simulink model "Potoo_Dyn_Model_v3px4_Flap_compact"  (R2024b)
settings: Solver=FixedStepAuto  StartTime=0.0  StopTime=120  FixedStep=0.001  MaxStep=0.001  RelTol=1e-3
InitFcn:
  | Tmech = 0.004;
undefined symbols (not defined in the file): Control, custom_ff, DiscIntNeverNeededParam, Earth, F, fractalcoef, Light, MIL, Potoo, Px4_Parms, realflap, tau, theta_max, thetadot_max, WGS84
libraries: cstblocks x10, matrix_library x10, aerolibasang x7, simulink x6, aerolibadyn x3, sharedtransform x2, slctrl_autotuning x1, mspfiltlib x1, mspsensorlib x1, shared6dof x1, aerolibactuator x1, aerolibatmos2 x1
(part 1 of 2)
settings Model: Creator=antho  LastModifiedBy=Nathan
settings SolverCC: AutoInsertRateTranBlk=on

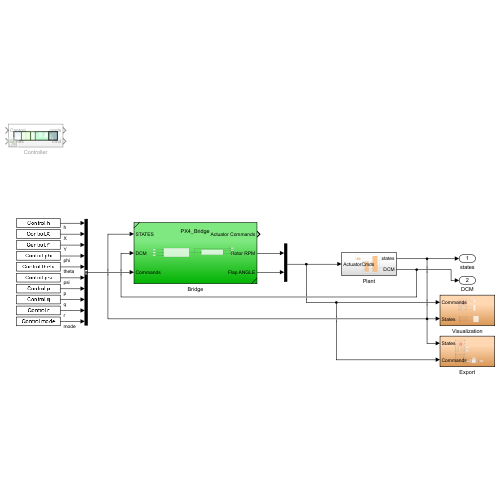
[thumbnail: Simulink's stored preview of the top-level diagram]
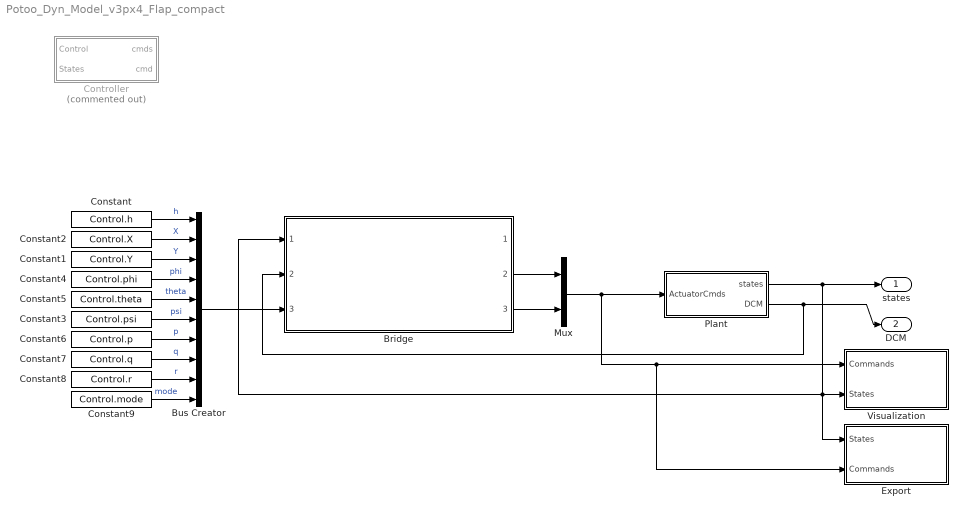
== system Potoo_Dyn_Model_v3px4_Flap_compact ==
  Bridge : Subsystem  ReferencedSubsystem=PX4_Bridge
  Bus Creator : BusCreator  Inputs=10
  Constant : Constant  Value=Control.h
  Constant1 : Constant  Value=Control.Y
  Constant2 : Constant  Value=Control.X
  Constant3 : Constant  Value=Control.psi
  Constant4 : Constant  Value=Control.phi
  Constant5 : Constant  Value=Control.theta
  Constant6 : Constant  Value=Control.p
  Constant7 : Constant  Value=Control.q
  Constant8 : Constant  Value=Control.r
  Constant9 : Constant  Value=Control.mode
  Controller : Subsystem  Commented=on
  Export : Subsystem
  Mux : Mux  Inputs=2
  Plant : Subsystem
  Visualization : Subsystem
  states : Outport
  DCM : Outport  Port=2
  wires:
  Plant/1(states) -> Bridge/1, Visualization/2(States), Export/1(States), states/1
  Plant/2(DCM) -> Bridge/2, DCM/1
  Constant/1 -> Bus Creator/1  "h"
  Constant2/1 -> Bus Creator/2  "X"
  Constant1/1 -> Bus Creator/3  "Y"
  Mux/1 -> Plant/1(ActuatorCmds), Export/2(Commands), Visualization/1(Commands)
  Bus Creator/1 -> Bridge/3
  Constant4/1 -> Bus Creator/4  "phi"
  Constant5/1 -> Bus Creator/5  "theta"
  Constant3/1 -> Bus Creator/6  "psi"
  Constant6/1 -> Bus Creator/7  "p"
  Constant7/1 -> Bus Creator/8  "q"
  Constant8/1 -> Bus Creator/9  "r"
  Constant9/1 -> Bus Creator/10  "mode"
  Bridge/3 -> Mux/2
  Bridge/2 -> Mux/1

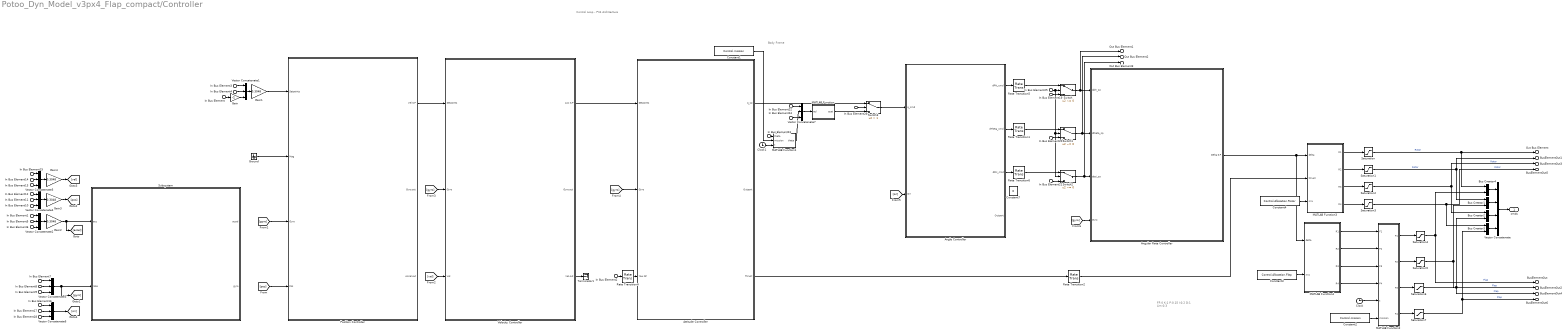
== system Potoo_Dyn_Model_v3px4_Flap_compact/Controller ==
  note: FF:0
      | K:1
      | P:0.15
      | I:0.2
      | D:1
      | Lim:0.3
  note: Control Loop - PX4 Architecture
  note: Body Frame
  In Bus Element : Inport  PortName=Control  Element=h
  In Bus Element2 : Inport  PortName=Control  Element=psi
  In Bus Element24 : Inport  PortName=Control  Element=psi
  In Bus Element3 : Inport  PortName=Control  Element=X
  In Bus Element4 : Inport  PortName=Control  Element=Y
  In Bus Element19 : Inport  PortName=Control  Element=p
  In Bus Element20 : Inport  PortName=Control  Element=q
  In Bus Element21 : Inport  PortName=Control  Element=r
  In Bus Element22 : Inport  PortName=Control  Element=phi
  In Bus Element23 : Inport  PortName=Control  Element=theta
  In Bus Element25 : Inport  PortName=Control  Element=mode
  In Bus Element26 : Inport  PortName=Control  Element=mode
  In Bus Element1 : Inport  Port=2  PortName=States  Element=Axe
  In Bus Element5 : Inport  Port=2  PortName=States  Element=Aye
  In Bus Element6 : Inport  Port=2  PortName=States  Element=Aze
  In Bus Element7 : Inport  Port=2  PortName=States  Element=p
  In Bus Element8 : Inport  Port=2  PortName=States  Element=q
  In Bus Element9 : Inport  Port=2  PortName=States  Element=r
  In Bus Element12 : Inport  Port=2  PortName=States  Element=Xe
  In Bus Element11 : Inport  Port=2  PortName=States  Element=Ye
  In Bus Element10 : Inport  Port=2  PortName=States  Element=Ze
  In Bus Element15 : Inport  Port=2  PortName=States  Element=Vxe
  In Bus Element14 : Inport  Port=2  PortName=States  Element=Vye
  In Bus Element13 : Inport  Port=2  PortName=States  Element=Vze
  In Bus Element16 : Inport  Port=2  PortName=States  Element=phi
  In Bus Element17 : Inport  Port=2  PortName=States  Element=theta
  In Bus Element18 : Inport  Port=2  PortName=States  Element=psi
  Angle Controller : Subsystem  mask{MC_ROLL_P=Px4_Parms.MC_ROLL_P, MC_PITCH_P=Px4_Parms.MC_PITCH_P, MC_YAW_P=Px4_Parms.MC_YAW_P, MC_ROLLRATE_MAX=Px4_Parms.MC_ROLLRATE_MAX, MC_PITCHRATE_MAX=Px4_Parms.MC_PITCHRATE_MAX, MC_YAWRATE_MAX=Px4_Parms.MC_YAWRATE_MAX, MC_ACRO_R_MAX=Px4_Parms.MC_ACRO_R_MAX, MC_YAW_WEIGHT=Px4_Parms.MC_YAW_WEIGHT, m=Px4_Parms.m}
      mask prompts: MC_ROLL_P "MC_ROLL_P ="; MC_PITCH_P "MC_PITCH_P ="; MC_YAW_P "MC_YAW_P ="; MC_ROLLRATE_MAX "MC_ROLLRATE_MAX ="; MC_PITCHRATE_MAX "MC_PITCHRATE_MAX ="; MC_YAWRATE_MAX "MC_YAWRATE_MAX ="; MC_ACRO_R_MAX "MC_ACRO_R_MAX ="; MC_YAW_WEIGHT "MC_YAW_WEIGHT ="; m "m [kg] ="
      mask DialogControl DescTextVar Prompt: Attitude Controller - based on PX4 architecture
      mask Display:
      | disp('Angle Control')
      | 
      | port_label('input',1,'q_{sp}','texmode','on')
      | port_label('input',2,'Gyro')
      | 
      | port_label('output',1,'d\phi_{cmd}','texmode','on')
      | port_label('output',2,'d\theta_{cmd}','texmode','on')
      | port_label('output',3,'d\psi_{cmd}','texmode','on')
      | port_label('output',4,'Gyro','texmode','on')
  Angular Rate Controller : Subsystem  mask{MC_ROLLRATE_FF=Px4_Parms.MC_ROLLRATE_FF, MC_ROLLRATE_K=Px4_Parms.MC_ROLLRATE_K, MC_ROLLRATE_P=Px4_Parms.MC_ROLLRATE_P, MC_ROLLRATE_I=Px4_Parms.MC_ROLLRATE_I, MC_ROLLRATE_D=Px4_Parms.MC_ROLLRATE_D, MC_RR_INT_LIM=Px4_Parms.MC_RR_INT_LIM, MC_PITCHRATE_FF=Px4_Parms.MC_PITCHRATE_FF, MC_PITCHRATE_K=Px4_Parms.MC_PITCHRATE_K, MC_PITCHRATE_P=Px4_Parms.MC_PITCHRATE_P, MC_PITCHRATE_I=Px4_Parms.MC_PITCHRATE_I, MC_PITCHRATE_D=Px4_Parms.MC_PITCHRATE_D, MC_PR_INT_LIM=Px4_Parms.MC_PR_INT_LIM, MC_YAWRATE_K=Px4_Parms.MC_YAWRATE_K, MC_YAWRATE_P=Px4_Parms.MC_YAWRATE_P, MC_YAWRATE_I=Px4_Parms.MC_YAWRATE_I, MC_YAWRATE_D=Px4_Parms.MC_YAWRATE_D, MC_YR_INT_LIM=Px4_Parms.MC_YR_INT_LIM, IMU_DGYRO_CUTOFF=Px4_Parms.IMU_DGYRO_CUTOFF, IMU_GYRO_CUTOFF=Px4_Parms.IMU_GYRO_CUTOFF}
      mask prompts: MC_ROLLRATE_FF "MC_ROLLRATE_FF ="; MC_ROLLRATE_K "MC_ROLLRATE_K ="; MC_ROLLRATE_P "MC_ROLLRATE_P ="; MC_ROLLRATE_I "MC_ROLLRATE_I ="; MC_ROLLRATE_D "MC_ROLLRATE_D ="; MC_RR_INT_LIM "MC_RR_INT_LIM ="; MC_PITCHRATE_FF "MC_PITCHRATE_FF ="; MC_PITCHRATE_K "MC_PITCHRATE_K ="; MC_PITCHRATE_P "MC_PITCHRATE_P ="; MC_PITCHRATE_I "MC_PITCHRATE_I ="; MC_PITCHRATE_D "MC_PITCHRATE_D ="; MC_PR_INT_LIM "MC_PR_INT_LIM ="; MC_YAWRATE_K "MC_YAWRATE_K ="; MC_YAWRATE_P "MC_YAWRATE_P ="; MC_YAWRATE_I "MC_YAWRATE_I ="; MC_YAWRATE_D "MC_YAWRATE_D ="; MC_YR_INT_LIM "MC_YR_INT_LIM ="; IMU_DGYRO_CUTOFF "IMU_DGYRO_CUTOFF ="; IMU_GYRO_CUTOFF "IMU_GYRO_CUTOFF ="
      mask DialogControl DescTextVar Prompt: Angular rate controller, based on PX4 architecture
      mask DialogControl ROLL Prompt: Roll
      mask DialogControl PITCH Prompt: Pitch
      mask DialogControl YAW Prompt: Yaw
      mask Display:
      | disp('Angular Rate Controller')
      | 
      | port_label('input',1,'d\phi_{cmd}','texmode','on')
      | port_label('input',2,'d\theta_{cmd}','texmode','on')
      | port_label('input',3,'d\psi_{cmd}','texmode','on')
      | port_label('input',4,'Gyro','texmode','on')
      | 
      | port_label('output',1,'\delta_{cmd}','texmode','on')
  Attitude Controller : Subsystem  mask{MC_ROLL_P=Px4_Parms.MC_ROLL_P, MC_PITCH_P=Px4_Parms.MC_PITCH_P, MC_YAW_P=Px4_Parms.MC_YAW_P, MC_ROLLRATE_MAX=Px4_Parms.MC_ROLLRATE_MAX, MC_PITCHRATE_MAX=Px4_Parms.MC_PITCHRATE_MAX, MC_YAWRATE_MAX=Px4_Parms.MC_YAWRATE_MAX, MC_ACRO_R_MAX=Px4_Parms.MC_ACRO_R_MAX, MC_YAW_WEIGHT=Px4_Parms.MC_YAW_WEIGHT, m=Px4_Parms.m}
      mask prompts: MC_ROLL_P "MC_ROLL_P ="; MC_PITCH_P "MC_PITCH_P ="; MC_YAW_P "MC_YAW_P ="; MC_ROLLRATE_MAX "MC_ROLLRATE_MAX ="; MC_PITCHRATE_MAX "MC_PITCHRATE_MAX ="; MC_YAWRATE_MAX "MC_YAWRATE_MAX ="; MC_ACRO_R_MAX "MC_ACRO_R_MAX ="; MC_YAW_WEIGHT "MC_YAW_WEIGHT ="; m "m [kg] ="
      mask DialogControl DescTextVar Prompt: Attitude Controller - based on PX4 architecture
      mask Display:
      | disp('Attitude Controller')
      | 
      | port_label('input',1,'ACCEL. S.P')
      | port_label('input',2,'Gyro')
      | port_label('input',3,'\psi_{cmd}','texmode','on')
      | 
      | port_label('output',1,'q_{sp}','texmode','on')
      | port_label('output',2,'Gyro','texmode','on')
      | port_label('output',3,'Thrust_{cmd}','texmode','on')
  Bus Creator{1..4} (4 alike) : BusCreator  Inputs=2  OutDataTypeStr=Bus: ActuatorCmds  NonVirtualBus=on
  Clock : Clock
  Clock1 : Clock
  Constant1 : Constant  Value=Control.mission  VectorParams1D=off
  Constant2 : Constant  Value=Control.mission  VectorParams1D=off
  Constant3 : Constant  Value=Control.Allocation.Flap  VectorParams1D=off
  Constant4 : Constant  Value=Control.Allocation.Rotor  VectorParams1D=off
  Constant7 : Constant  Value=0
  Gain : Gain  Gain=-1
  Gain{1..4} (4 alike) : Gain  Gain=0.3048
  Ground : Ground
  MATLAB Function : MATLAB Function  TreatAsAtomicUnit=on
  MATLAB Function1 : MATLAB Function  TreatAsAtomicUnit=on
  MATLAB Function2 : MATLAB Function  TreatAsAtomicUnit=on
  MATLAB Function3 : MATLAB Function  TreatAsAtomicUnit=on
  MATLAB Function4 : MATLAB Function  TreatAsAtomicUnit=on
  Position Controller : Subsystem  mask{MPC_XY_P=Px4_Parms.MPC_XY_P, MPC_XY_VEL_MAX=Px4_Parms.MPC_XY_VEL_MAX, MPC_Z_P=Px4_Parms.MPC_Z_P, MPC_Z_VEL_MAX_UP=Px4_Parms.MPC_Z_VEL_MAX_UP, MPC_Z_VEL_MAX_DOWN=Px4_Parms.MPC_Z_VEL_MAX_DOWN}
      mask prompts: MPC_XY_P "MPC_XY_P ="; MPC_XY_VEL_MAX "MPC_XY_VEL_MAX ="; MPC_Z_P "MPC_Z_P ="; MPC_Z_VEL_MAX_UP "MPC_Z_VEL_MAX_UP ="; MPC_Z_VEL_MAX_DOWN "MPC_Z_VEL_MAX_DOWN ="
      mask DialogControl DescTextVar Prompt: Position Controller - based on PX4 architecture
      mask Display:
      | disp('Position Controller')
      | 
      | port_label('input',1,'POS. S.P')
      | port_label('input',4,'Accel')
      | port_label('input',3,'Gyro')
      | port_label('input',2,'Mag')
      | 
      | port_label('output',1,'VEL. S.P','texmode','on')
      | port_label('output',3,'Accel','texmode','on')
      | port_label('output',2,'Gyro','texmode','on')
  Rate Transition{1..2,5..6} (4 alike) : RateTransition  OutPortSampleTime=1/1000
  Rate Transition4 : RateTransition  OutPortSampleTime=1/ 250
  Saturation{,1..3} (4 alike) : Saturate  UpperLimit=8000  LowerLimit=0
  Saturation{4..7} (4 alike) : Saturate  UpperLimit=20  LowerLimit=-20
  Subsystem : Subsystem
      mask Display:
      | disp('IMU + AHRS')
      | port_label('input',1,'Acceleration','texmode','on')
      | port_label('input',2,'Angular rate','texmode','on')
      | port_label('output',2,'Gyroscope','texmode','on')
      | port_label('output',1,'Accelometer','texmode','on')
  Switch : Switch  Criteria=u2 ~= 0  SaturateOnIntegerOverflow=off  InputSameDT=off
  Switch1 : Switch  Criteria=u2 ~= 0  SaturateOnIntegerOverflow=off  InputSameDT=off
  Switch2 : Switch  Criteria=u2 ~= 0  SaturateOnIntegerOverflow=off  InputSameDT=off
  Switch3 : Switch  Criteria=u2 > Threshold  Threshold=1  SaturateOnIntegerOverflow=off  InputSameDT=off
  Terminator1 : Terminator
  Vector Concatenate : Concatenate  NumInputs=4
  Vector Concatenate{1..7} (7 alike) : Concatenate  NumInputs=3
  Velocity Controller : Subsystem  mask{MPC_XY_VEL_P_ACC=Px4_Parms.MPC_XY_VEL_P_ACC, MPC_XY_VEL_I_ACC=Px4_Parms.MPC_XY_VEL_I_ACC, MPC_XY_VEL_D_ACC=Px4_Parms.MPC_XY_VEL_D_ACC, MPC_Z_VEL_P_ACC=Px4_Parms.MPC_Z_VEL_P_ACC, MPC_Z_VEL_I_ACC=Px4_Parms.MPC_Z_VEL_I_ACC, MPC_Z_VEL_D_ACC=Px4_Parms.MPC_Z_VEL_D_ACC, MPC_VELD_LP=Px4_Parms.MPC_VELD_LP, MPC_TILTMAX_AIR=Px4_Parms.MPC_TILTMAX_AIR, MPC_THR_MAX=Px4_Parms.MPC_THR_MAX}
      mask prompts: MPC_XY_VEL_P_ACC "MPC_XY_VEL_P_ACC ="; MPC_XY_VEL_I_ACC "MPC_XY_VEL_I_ACC ="; MPC_XY_VEL_D_ACC "MPC_XY_VEL_D_ACC ="; MPC_Z_VEL_P_ACC "MPC_Z_VEL_P_ACC ="; MPC_Z_VEL_I_ACC "MPC_Z_VEL_I_ACC ="; MPC_Z_VEL_D_ACC "MPC_Z_VEL_D_ACC ="; MPC_VELD_LP "MPC_VELD_LP ="; MPC_TILTMAX_AIR "MPC_TILTMAX_AIR ="; MPC_THR_MAX "MPC_THR_MAX ="
      mask DialogControl DescTextVar Prompt: Velocity Controller - based on PX4 architecture
      mask DialogControl Container3 Prompt: XY -  Velocity
      mask DialogControl Container4 Prompt: Z - Velocity
      mask DialogControl Container5 Prompt: General Parameters
      mask Display:
      | disp('Velocity Controller')
      | 
      | port_label('input',1,'VEL. S.P')
      | port_label('input',3,'Accel')
      | port_label('input',2,'Gyro')
      | 
      | port_label('output',1,'ACCEL. S.P','texmode','on')
      | port_label('output',3,'Accel','texmode','on')
      | port_label('output',2,'Gyro','texmode','on')
  cmds : Outport
  Out Bus Element : Outport  Port=2  PortName=cmd  Element=Rotor1
  BusElementOut : Outport  Port=2  PortName=cmd  Element=Flap1
  BusElementOut1 : Outport  Port=2  PortName=cmd  Element=Rotor2
  BusElementOut2 : Outport  Port=2  PortName=cmd  Element=Flap2
  BusElementOut3 : Outport  Port=2  PortName=cmd  Element=Rotor3
  BusElementOut4 : Outport  Port=2  PortName=cmd  Element=Flap3
  BusElementOut5 : Outport  Port=2  PortName=cmd  Element=Rotor4
  BusElementOut6 : Outport  Port=2  PortName=cmd  Element=Flap4
  Out Bus Element1 : Outport  Port=2  PortName=cmd  Element=p
  Out Bus Element2 : Outport  Port=2  PortName=cmd  Element=q
  Out Bus Element3 : Outport  Port=2  PortName=cmd  Element=r
  wires:
  Saturation1/1 -> Bus Creator1/1, BusElementOut1/1  "Rotor"
  Saturation3/1 -> BusElementOut5/1, Bus Creator3/1  "Rotor"
  Saturation/1 -> Bus Creator4/1, Out Bus Element/1  "Rotor"
  Saturation2/1 -> BusElementOut3/1, Bus Creator2/1  "Rotor"
  Saturation4/1 -> BusElementOut/1, Bus Creator4/2  "Flap"
  Saturation6/1 -> BusElementOut4/1, Bus Creator2/2  "Flap"
  Saturation7/1 -> Bus Creator3/2, BusElementOut6/1  "Flap"
  Clock/1 -> MATLAB Function2/5(t)
  MATLAB Function2/4(F4) -> Saturation7/1
  MATLAB Function2/3(F3) -> Saturation6/1
  MATLAB Function2/2(F2) -> Saturation5/1
  MATLAB Function2/1(F1) -> Saturation4/1
  Bus Creator4/1 -> Vector Concatenate/1
  Bus Creator1/1 -> Vector Concatenate/2
  Bus Creator2/1 -> Vector Concatenate/3
  Bus Creator3/1 -> Vector Concatenate/4
  Saturation5/1 -> BusElementOut2/1, Bus Creator1/2  "Flap"
  Vector Concatenate/1 -> cmds/1
  Constant2/1 -> MATLAB Function2/6(mission)
  Constant4/1 -> MATLAB Function3/3(mix)
  In Bus Element2/1 -> Rate Transition4/1
  In Bus Element/1 -> Gain/1
  Vector Concatenate3/1 -> Subsystem/2(rate), [gyro]
  In Bus Element6/1 -> Vector Concatenate2/3
  In Bus Element7/1 -> Vector Concatenate3/1
  In Bus Element8/1 -> Vector Concatenate3/2
  Gain/1 -> Vector Concatenate1/3
  Ground/1 -> Position Controller/2(Mag)
  In Bus Element9/1 -> Vector Concatenate3/3
  Angle Controller/3(dPsi_cmd) -> Rate Transition6/1
  Attitude Controller/3(Thrust) -> Rate Transition2/1
  Vector Concatenate1/1 -> Gain1/1
  Angle Controller/1(dPhi_cmd) -> Rate Transition5/1
  In Bus Element5/1 -> Vector Concatenate2/2
  Velocity Controller/1(Acc S.P) -> Attitude Controller/1(Setpoints)
  In Bus Element3/1 -> Vector Concatenate1/1
  Gain1/1 -> Position Controller/1(Setpoints)
  Angle Controller/2(dTheta_cmd) -> Rate Transition1/1
  [gyro] -> Angular Rate Controller/4(Gyro)
  Vector Concatenate2/1 -> Gain2/1
  In Bus Element1/1 -> Vector Concatenate2/1
  Velocity Controller/3(Vel.out) -> Terminator1/1
  Rate Transition4/1 -> Attitude Controller/3(Yaw.SP)
  In Bus Element4/1 -> Vector Concatenate1/2
  Constant3/1 -> MATLAB Function4/2(mix)
  Gain2/1 -> Subsystem/1(acc), [accel]
  MATLAB Function3/1(R1) -> Saturation/1
  MATLAB Function3/2(R2) -> Saturation1/1
  MATLAB Function3/3(R3) -> Saturation2/1
  MATLAB Function3/4(R4) -> Saturation3/1
  MATLAB Function4/1(R1) -> MATLAB Function2/1("F1 ")
  MATLAB Function4/2(R2) -> MATLAB Function2/2("F2 ")
  MATLAB Function4/3(R3) -> MATLAB Function2/3("F3 ")
  MATLAB Function4/4(R4) -> MATLAB Function2/4("F4 ")
  Rate Transition2/1 -> MATLAB Function3/2(thrust)
  [pos] -> Position Controller/4(Pos)
  [gyro] -> Position Controller/3(Gyro)
  In Bus Element11/1 -> Vector Concatenate4/2
  In Bus Element12/1 -> Vector Concatenate4/1
  In Bus Element10/1 -> Vector Concatenate4/3
  Vector Concatenate4/1 -> Gain3/1
  Gain3/1 -> [pos]
  In Bus Element15/1 -> Vector Concatenate5/1
  In Bus Element14/1 -> Vector Concatenate5/2
  In Bus Element13/1 -> Vector Concatenate5/3
  Vector Concatenate5/1 -> Gain4/1
  Gain4/1 -> [vel]
  [vel] -> Velocity Controller/3(Vel)
  [gyro] -> Velocity Controller/2(Gyro)
  In Bus Element16/1 -> Vector Concatenate6/1
  In Bus Element17/1 -> Vector Concatenate6/2
  In Bus Element18/1 -> Vector Concatenate6/3
  Vector Concatenate6/1 -> [ori]
  [gyro] -> Attitude Controller/2(Gyro)
  [ori] -> Angle Controller/2(Ori)
  In Bus Element25/1 -> Switch2/2, Switch1/2, Switch/2
  Switch/1 -> Out Bus Element1/1, Angular Rate Controller/1(dphi_sp)
  Switch1/1 -> Angular Rate Controller/2(dtheta_sp), Out Bus Element2/1
  Switch2/1 -> Out Bus Element3/1, Angular Rate Controller/3(dpsi_sp)
  Rate Transition5/1 -> Switch/1
  Rate Transition6/1 -> Switch2/1
  In Bus Element26/1 -> Switch3/2
  Attitude Controller/1(q_sp) -> Switch3/1
  Switch3/1 -> Angle Controller/1(q_cmd)
  MATLAB Function/1(quat) -> Switch3/3
  Vector Concatenate7/1 -> MATLAB Function/1(eul)
  In Bus Element19/1 -> Switch/3
  In Bus Element22/1 -> Vector Concatenate7/1
  In Bus Element21/1 -> Switch2/3
  In Bus Element24/1 -> Vector Concatenate7/3
  Rate Transition1/1 -> Switch1/1
  Position Controller/1(Vel S.P) -> Velocity Controller/1(Setpoints)
  Angular Rate Controller/1(Delta S.P) -> MATLAB Function4/1(delta), MATLAB Function3/1(delta)
  In Bus Element20/1 -> Switch1/3
  In Bus Element23/1 -> MATLAB Function1/1("theta ")
  MATLAB Function1/1(theta) -> Vector Concatenate7/2
  Clock1/1 -> MATLAB Function1/3(t)
  Constant1/1 -> MATLAB Function1/2(mission)

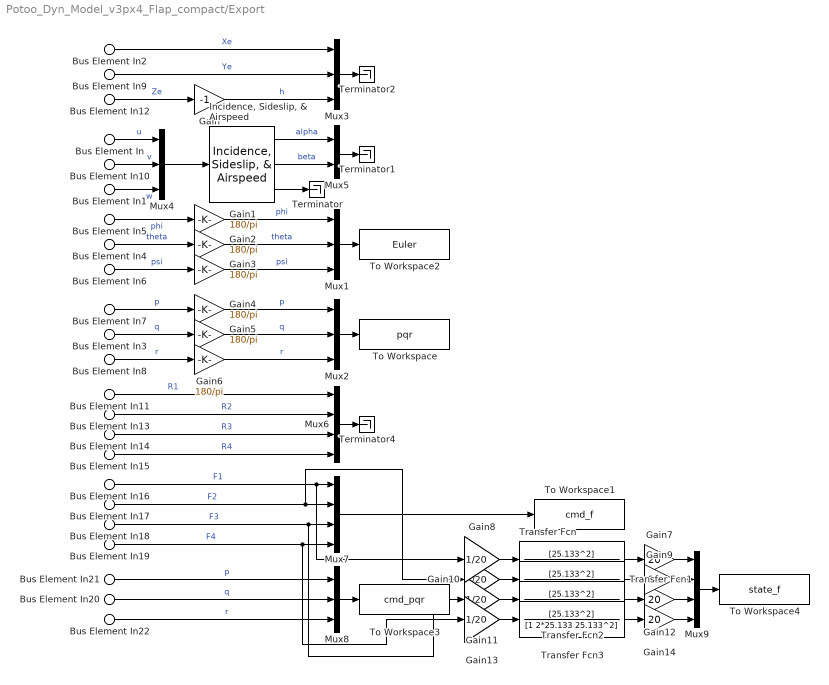
== system Potoo_Dyn_Model_v3px4_Flap_compact/Export ==
  Bus Element In : Inport  PortName=States  Element=u
  Bus Element In1 : Inport  PortName=States  Element=w
  Bus Element In3 : Inport  PortName=States  Element=q
  Bus Element In4 : Inport  PortName=States  Element=theta
  Bus Element In12 : Inport  PortName=States  Element=Ze
  Bus Element In2 : Inport  PortName=States  Element=Xe
  Bus Element In10 : Inport  PortName=States  Element=v
  Bus Element In5 : Inport  PortName=States  Element=phi
  Bus Element In6 : Inport  PortName=States  Element=psi
  Bus Element In7 : Inport  PortName=States  Element=p
  Bus Element In8 : Inport  PortName=States  Element=r
  Bus Element In9 : Inport  PortName=States  Element=Ye
  Bus Element In11 : Inport  Port=2  PortName=Commands  Element=Rotor1
  Bus Element In13 : Inport  Port=2  PortName=Commands  Element=Rotor2
  Bus Element In14 : Inport  Port=2  PortName=Commands  Element=Rotor3
  Bus Element In15 : Inport  Port=2  PortName=Commands  Element=Rotor4
  Bus Element In16 : Inport  Port=2  PortName=Commands  Element=Flap1
  Bus Element In17 : Inport  Port=2  PortName=Commands  Element=Flap2
  Bus Element In18 : Inport  Port=2  PortName=Commands  Element=Flap3
  Bus Element In19 : Inport  Port=2  PortName=Commands  Element=Flap4
  Bus Element In20 : Inport  Port=2  PortName=Commands  Element=q
  Bus Element In21 : Inport  Port=2  PortName=Commands  Element=p
  Bus Element In22 : Inport  Port=2  PortName=Commands  Element=r
  Gain : Gain  Gain=-1
  Gain{1..6} (6 alike) : Gain  Gain=180/pi
  Gain{8,10..11,13} (4 alike) : Gain  Gain=1/20
  Gain{7,9,12,14} (4 alike) : Gain  Gain=20
  "Incidence, Sideslip, & Airspeed" : aerolibasang/Incidence, Sideslip, & Airspeed
  Mux{1..4,8} (5 alike) : Mux  Inputs=3
  Mux5 : Mux  Inputs=2
  Mux6 : Mux
  Mux7 : Mux
  Mux9 : Mux
  Terminator{,1..2,4} (4 alike) : Terminator
  To Workspace : ToWorkspace  VariableName=pqr  SaveFormat=Structure With Time  SampleTime=-1
  To Workspace1 : ToWorkspace  VariableName=cmd_f  SaveFormat=Structure With Time  SampleTime=-1
  To Workspace2 : ToWorkspace  VariableName=Euler  SaveFormat=Structure With Time  SampleTime=-1
  To Workspace3 : ToWorkspace  VariableName=cmd_pqr  SaveFormat=Structure With Time  SampleTime=-1
  To Workspace4 : ToWorkspace  VariableName=state_f  SaveFormat=Structure With Time  SampleTime=-1
  Transfer Fcn{,1..3} (4 alike) : TransferFcn  Numerator=[25.133^2]  Denominator=[1 2*25.133 25.133^2]
  wires:
  Gain6/1 -> Mux2/3  "r"
  Gain5/1 -> Mux2/2  "q"
  Gain4/1 -> Mux2/1  "p"
  Gain3/1 -> Mux1/3  "psi"
  Gain2/1 -> Mux1/2  "theta"
  Gain1/1 -> Mux1/1  "phi"
  Gain/1 -> Mux3/3  "h"
  Mux5/1 -> Terminator1/1
  "Incidence, Sideslip, & Airspeed"/3 -> Terminator/1
  Bus Element In/1 -> Mux4/1  "u"
  Bus Element In1/1 -> Mux4/3  "w"
  Bus Element In3/1 -> Gain5/1  "q"
  Bus Element In4/1 -> Gain2/1  "theta"
  Bus Element In5/1 -> Gain1/1  "phi"
  Bus Element In6/1 -> Gain3/1  "psi"
  Bus Element In7/1 -> Gain4/1  "p"
  Bus Element In8/1 -> Gain6/1  "r"
  Bus Element In10/1 -> Mux4/2  "v"
  Mux4/1 -> "Incidence, Sideslip, & Airspeed"/1
  "Incidence, Sideslip, & Airspeed"/1 -> Mux5/1  "alpha"
  "Incidence, Sideslip, & Airspeed"/2 -> Mux5/2  "beta"
  Bus Element In12/1 -> Gain/1  "Ze"
  Bus Element In9/1 -> Mux3/2  "Ye"
  Bus Element In2/1 -> Mux3/1  "Xe"
  Mux1/1 -> To Workspace2/1
  Mux3/1 -> Terminator2/1
  Mux6/1 -> Terminator4/1
  Mux2/1 -> To Workspace/1
  Mux7/1 -> To Workspace1/1
  Bus Element In14/1 -> Mux6/3  "R3"
  Bus Element In15/1 -> Mux6/4  "R4"
  Bus Element In13/1 -> Mux6/2  "R2"
  Bus Element In16/1 -> Gain8/1, Mux7/1  "F1"
  Bus Element In11/1 -> Mux6/1  "R1"
  Bus Element In18/1 -> Gain11/1, Mux7/3  "F3"
  Bus Element In19/1 -> Gain13/1, Mux7/4  "F4"
  Bus Element In17/1 -> Gain10/1, Mux7/2  "F2"
  Bus Element In20/1 -> Mux8/2  "q"
  Bus Element In21/1 -> Mux8/1  "p"
  Bus Element In22/1 -> Mux8/3  "r"
  Mux8/1 -> To Workspace3/1
  Transfer Fcn/1 -> Gain7/1
  Gain8/1 -> Transfer Fcn/1
  Gain7/1 -> Mux9/1
  Mux9/1 -> To Workspace4/1
  Gain10/1 -> Transfer Fcn1/1
  Transfer Fcn1/1 -> Gain9/1
  Gain9/1 -> Mux9/2
  Transfer Fcn2/1 -> Gain12/1
  Gain11/1 -> Transfer Fcn2/1
  Gain12/1 -> Mux9/3
  Gain13/1 -> Transfer Fcn3/1
  Transfer Fcn3/1 -> Gain14/1
  Gain14/1 -> Mux9/4

== system Potoo_Dyn_Model_v3px4_Flap_compact/Plant ==
  ActuatorCmds : Inport
  6DOF EOM : Subsystem  VariantControl=eom3DOF
  Aerodynamic Model : Subsystem  VariantControl=aeroCONST
  Environment Model : Subsystem  mask(Environment Model){spec=MIL-F-8785C, model=Continuous Dryden (+q -r), W20=5, Wdeg=0, TurbProb=10^-2 - Light, L_high=533.4, Wingspan=4, ts=0.1, Seed=[23341 23342 23343 23344], T_on=off, refAlt=0}
      mask prompts: spec "aeroblks:aeroblkwind:blockWindTurbulenceModelParamSpecification"; model "aeroblks:aeroblkwind:blockWindTurbulenceModelParamModeltype"; W20 "Wind speed at 6 m defines the low-altitude intensity (m/s):"; Wdeg "Wind direction at 6 m (degrees clockwise from north):"; TurbProb "aeroblks:aeroblkwind:blockWindTurbulenceModelParamProbabilityofexceedanceofhighaltitudeintensity"; L_high "Scale length at medium/high altitudes (m):"; Wingspan "Wingspan (m):"; ts "Band limited noise sample time (sec):"; Seed "aeroblks:aeroblkwind:blockWindTurbulenceModelParamNoiseseedsugvgwgpg"; T_on "aeroblks:aeroblkwind:blockWindTurbulenceModelParamTurbulenceon"; refAlt "Reference height from Earth's surface to Flat Earth frame [m]:"
      mask help: This block contains an athmospheric model, a wind turbulence model, and a gravity model.
      mask Help: helpview(fullfile(docroot,'toolbox','aeroblks','aeroblks.map'), 'environment1');
      mask TypeOptions spec:
      | Dryden Wind Turbulence Model
      | (Continuous (+q +r))/spec
      mask TypeOptions model:
      | Dryden Wind Turbulence Model
      | (Continuous (+q +r))/model
      mask TypeOptions W20:
      | Dryden Wind Turbulence Model
      | (Continuous (+q +r))/W20
      mask TypeOptions Wdeg:
      | Dryden Wind Turbulence Model
      | (Continuous (+q +r))/Wdeg
      mask TypeOptions TurbProb:
      | Dryden Wind Turbulence Model
      | (Continuous (+q +r))/TurbProb
      mask TypeOptions L_high:
      | Dryden Wind Turbulence Model
      | (Continuous (+q +r))/L_high
      mask TypeOptions Wingspan:
      | Dryden Wind Turbulence Model
      | (Continuous (+q +r))/Wingspan
      mask TypeOptions ts:
      | Dryden Wind Turbulence Model
      | (Continuous (+q +r))/ts
      mask TypeOptions Seed:
      | Dryden Wind Turbulence Model
      | (Continuous (+q +r))/Seed
      mask TypeOptions T_on:
      | Dryden Wind Turbulence Model
      | (Continuous (+q +r))/T_on
      mask DialogControl Container4 Prompt: Atmospheric Model
      mask DialogControl Container17 Prompt: 1976 COESA-extended U.S. Standard Atmospheric Model
      mask DialogControl Control6 Prompt: There are no modifiable parameters for COESA.
      mask DialogControl Container6 Prompt: Wind Model
      mask DialogControl Container16 Prompt: Dryden Wind Turbulence Model
      mask DialogControl spec Prompt: Specification:
      mask DialogControl model Prompt: Model type:
      mask DialogControl TurbProb Prompt: Probability of exceedance of high-altitude intensity:
      mask DialogControl Seed Prompt: Noise seeds [ug vg wg pg]:
      mask DialogControl T_on Prompt: Turbulence on
      mask DialogControl Container8 Prompt: Gravity Model
      mask DialogControl Container18 Prompt: World Geodetic System (WGS 84) Gravity Taylor Series Model
      mask Display:
      | image('aeroenvironment.bmp',[.15,.15,.55,.75])
      | port_label('output',1,'Env')
  states : Outport
  DCM : Outport  Port=2
  wires:
  Environment Model/1(Env) -> Aerodynamic Model/1(Env), 6DOF EOM/1(Env)
  Aerodynamic Model/1(F) -> 6DOF EOM/2(Forces)
  Aerodynamic Model/2(M) -> 6DOF EOM/3(Moments)
  6DOF EOM/1(States) -> Aerodynamic Model/3(States), states/1, Environment Model/1(States)
  6DOF EOM/2(DCM) -> DCM/1
  ActuatorCmds/1 -> Aerodynamic Model/2(ActuatorCmds)

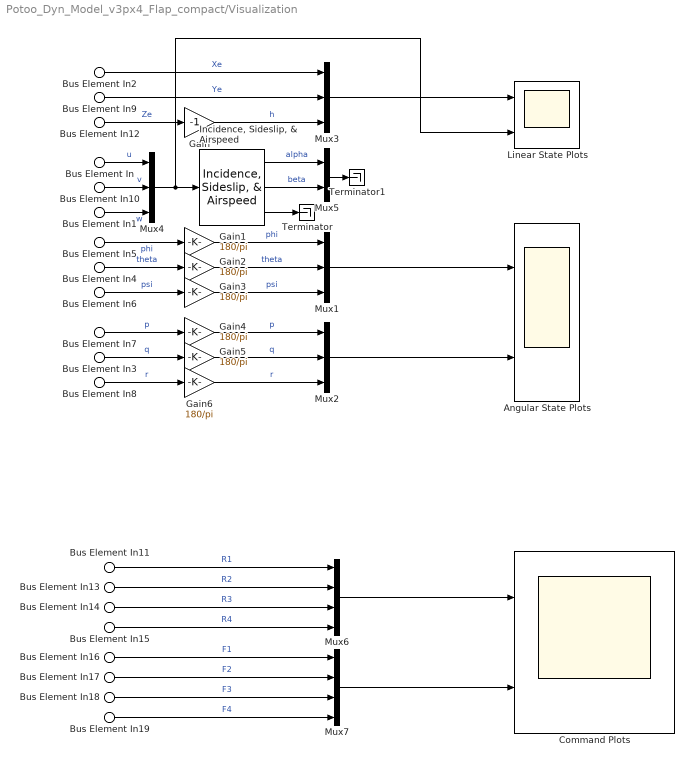
== system Potoo_Dyn_Model_v3px4_Flap_compact/Visualization ==
  Bus Element In11 : Inport  PortName=Commands  Element=Rotor1
  Bus Element In13 : Inport  PortName=Commands  Element=Rotor2
  Bus Element In14 : Inport  PortName=Commands  Element=Rotor3
  Bus Element In15 : Inport  PortName=Commands  Element=Rotor4
  Bus Element In16 : Inport  PortName=Commands  Element=Flap1
  Bus Element In17 : Inport  PortName=Commands  Element=Flap2
  Bus Element In18 : Inport  PortName=Commands  Element=Flap3
  Bus Element In19 : Inport  PortName=Commands  Element=Flap4
  Bus Element In : Inport  Port=2  PortName=States  Element=u
  Bus Element In1 : Inport  Port=2  PortName=States  Element=w
  Bus Element In3 : Inport  Port=2  PortName=States  Element=q
  Bus Element In4 : Inport  Port=2  PortName=States  Element=theta
  Bus Element In12 : Inport  Port=2  PortName=States  Element=Ze
  Bus Element In2 : Inport  Port=2  PortName=States  Element=Xe
  Bus Element In10 : Inport  Port=2  PortName=States  Element=v
  Bus Element In5 : Inport  Port=2  PortName=States  Element=phi
  Bus Element In6 : Inport  Port=2  PortName=States  Element=psi
  Bus Element In7 : Inport  Port=2  PortName=States  Element=p
  Bus Element In8 : Inport  Port=2  PortName=States  Element=r
  Bus Element In9 : Inport  Port=2  PortName=States  Element=Ye
  Angular State Plots : Scope  NumInputPorts=2
  Command Plots : Scope  NumInputPorts=2
  Gain : Gain  Gain=-1
  Gain{1..6} (6 alike) : Gain  Gain=180/pi
  "Incidence, Sideslip, & Airspeed" : aerolibasang/Incidence, Sideslip, & Airspeed
  Linear State Plots : Scope  NumInputPorts=2
  Mux{1..4} (4 alike) : Mux  Inputs=3
  Mux5 : Mux  Inputs=2
  Mux6 : Mux
  Mux7 : Mux
  Terminator : Terminator
  Terminator1 : Terminator
  wires:
  Mux3/1 -> Linear State Plots/1
  Bus Element In2/1 -> Mux3/1  "Xe"
  Bus Element In9/1 -> Mux3/2  "Ye"
  Bus Element In12/1 -> Gain/1  "Ze"
  Mux2/1 -> Angular State Plots/2
  Mux1/1 -> Angular State Plots/1
  "Incidence, Sideslip, & Airspeed"/2 -> Mux5/2  "beta"
  "Incidence, Sideslip, & Airspeed"/1 -> Mux5/1  "alpha"
  Mux4/1 -> Linear State Plots/2, "Incidence, Sideslip, & Airspeed"/1
  Bus Element In10/1 -> Mux4/2  "v"
  Bus Element In8/1 -> Gain6/1  "r"
  Bus Element In7/1 -> Gain4/1  "p"
  Bus Element In6/1 -> Gain3/1  "psi"
  Bus Element In5/1 -> Gain1/1  "phi"
  Bus Element In4/1 -> Gain2/1  "theta"
  Bus Element In3/1 -> Gain5/1  "q"
  Bus Element In1/1 -> Mux4/3  "w"
  Bus Element In/1 -> Mux4/1  "u"
  "Incidence, Sideslip, & Airspeed"/3 -> Terminator/1
  Mux5/1 -> Terminator1/1
  Gain/1 -> Mux3/3  "h"
  Gain1/1 -> Mux1/1  "phi"
  Gain2/1 -> Mux1/2  "theta"
  Gain3/1 -> Mux1/3  "psi"
  Gain4/1 -> Mux2/1  "p"
  Gain5/1 -> Mux2/2  "q"
  Gain6/1 -> Mux2/3  "r"
  Mux7/1 -> Command Plots/2
  Mux6/1 -> Command Plots/1
  Bus Element In14/1 -> Mux6/3  "R3"
  Bus Element In15/1 -> Mux6/4  "R4"
  Bus Element In13/1 -> Mux6/2  "R2"
  Bus Element In16/1 -> Mux7/1  "F1"
  Bus Element In11/1 -> Mux6/1  "R1"
  Bus Element In18/1 -> Mux7/3  "F3"
  Bus Element In19/1 -> Mux7/4  "F4"
  Bus Element In17/1 -> Mux7/2  "F2"

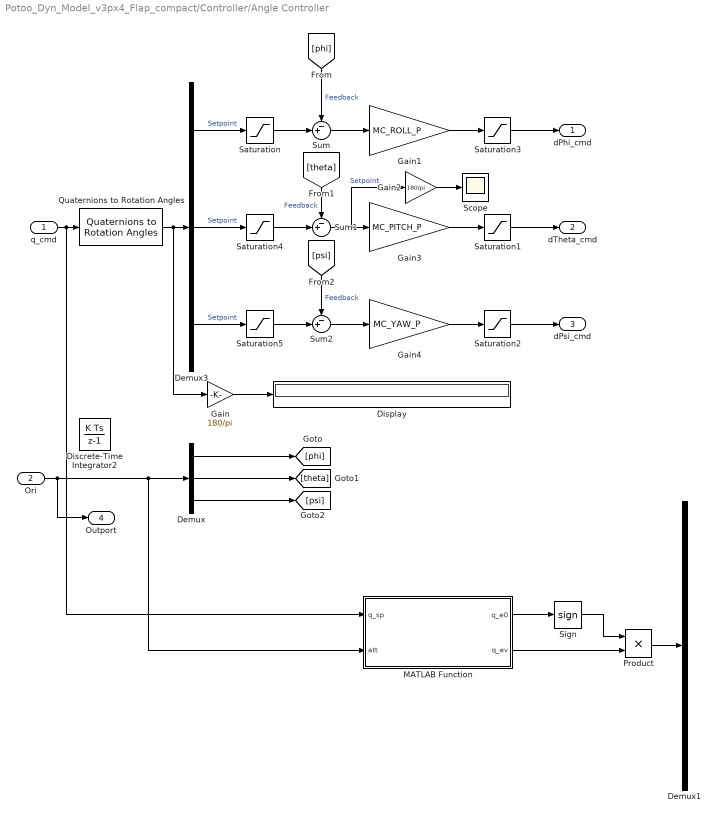
== system Potoo_Dyn_Model_v3px4_Flap_compact/Controller/Angle Controller ==
  q_cmd : Inport
  Ori : Inport  Port=2
  Demux : Demux  Outputs=3
  Demux1 : Demux  Outputs=3
  Demux3 : Demux  Outputs=3
  Discrete-Time Integrator2 : DiscreteIntegrator  InitialCondition=[0.001;0.001;0.001]  SampleTime=-1  ICPrevOutput=DiscIntNeverNeededParam  ICPrevScaledInput=DiscIntNeverNeededParam
  Display : Display
  Gain : Gain  Gain=180/pi
  Gain1 : Gain  Gain=MC_ROLL_P
  Gain2 : Gain  Gain=180/pi
  Gain3 : Gain  Gain=MC_PITCH_P
  Gain4 : Gain  Gain=MC_YAW_P
  MATLAB Function : MATLAB Function  TreatAsAtomicUnit=on
  Product : Product
  Quaternions to Rotation Angles : sharedtransform/Quaternions to Rotation Angles  rotationOrder=XYZ  aMode=aMode
  Saturation : Saturate  UpperLimit=1.5  LowerLimit=-1.5
  Saturation1 : Saturate  UpperLimit=MC_PITCHRATE_MAX  LowerLimit=-MC_PITCHRATE_MAX
  Saturation2 : Saturate  UpperLimit=MC_YAWRATE_MAX  LowerLimit=-MC_YAWRATE_MAX
  Saturation3 : Saturate  UpperLimit=MC_ROLLRATE_MAX  LowerLimit=-MC_ROLLRATE_MAX
  Saturation4 : Saturate  UpperLimit=1.5  LowerLimit=-1.5
  Saturation5 : Saturate  UpperLimit=1.5  LowerLimit=-1.5
  Scope : Scope
  Sign : Signum
  Sum : Sum  Inputs=-+|
  Sum1 : Sum  Inputs=-+|
  Sum2 : Sum  Inputs=-+|
  dPhi_cmd : Outport
  dTheta_cmd : Outport  Port=2
  dPsi_cmd : Outport  Port=3
  Outport : Outport  Port=4
  wires:
  Ori/1 -> MATLAB Function/2(att), Demux/1, Outport/1
  Demux/2 -> [theta]
  Demux/1 -> [phi]
  Demux/3 -> [psi]
  Demux3/1 -> Saturation/1  "Setpoint"
  Demux3/2 -> Saturation4/1  "Setpoint"
  Demux3/3 -> Saturation5/1  "Setpoint"
  Saturation3/1 -> dPhi_cmd/1
  Gain1/1 -> Saturation3/1
  Gain3/1 -> Saturation1/1
  Gain4/1 -> Saturation2/1
  Saturation1/1 -> dTheta_cmd/1
  Saturation2/1 -> dPsi_cmd/1
  [phi] -> Sum/1  "Feedback"
  [theta] -> Sum1/1  "Feedback"
  [psi] -> Sum2/1  "Feedback"
  q_cmd/1 -> Quaternions to Rotation Angles/1, MATLAB Function/1(q_sp)
  Saturation/1 -> Sum/2
  Saturation4/1 -> Sum1/2
  Saturation5/1 -> Sum2/2
  MATLAB Function/1(q_e0) -> Sign/1
  MATLAB Function/2(q_ev) -> Product/2
  Sign/1 -> Product/1
  Product/1 -> Demux1/1
  Sum/1 -> Gain1/1
  Sum1/1 -> Gain2/1, Gain3/1  "Setpoint"
  Sum2/1 -> Gain4/1
  Quaternions to Rotation Angles/1 -> Gain/1, Demux3/1
  Gain/1 -> Display/1
  Gain2/1 -> Scope/1

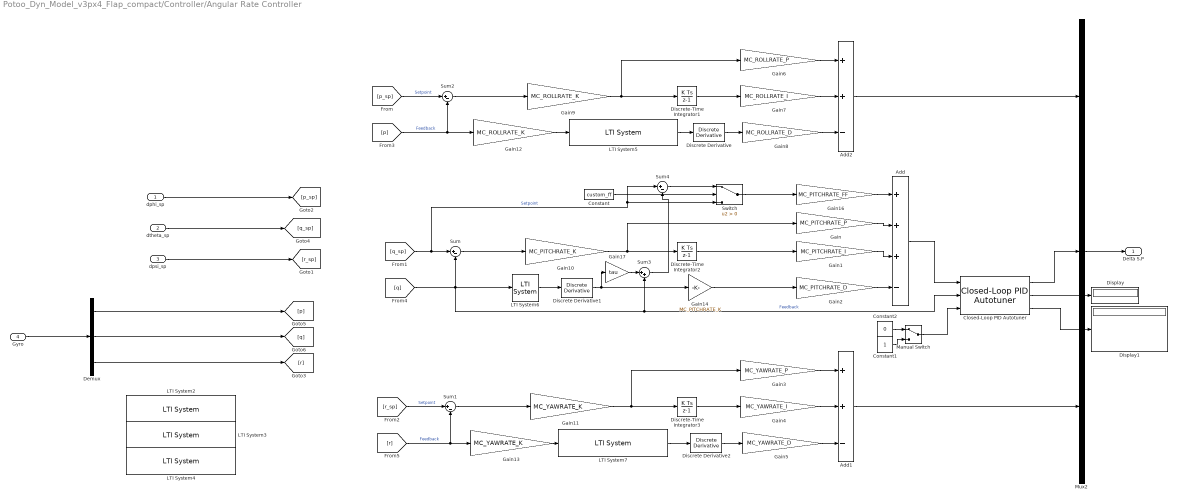
== system Potoo_Dyn_Model_v3px4_Flap_compact/Controller/Angular Rate Controller ==
  dphi_sp : Inport
  dtheta_sp : Inport  Port=2
  dpsi_sp : Inport  Port=3
  Gyro : Inport  Port=4
  Add : Sum  Inputs=+++-
  Add1 : Sum  Inputs=++-
  Add2 : Sum  Inputs=++-
  Closed-Loop PID Autotuner : slctrl_autotuning/Closed-Loop PID Autotuner  PIDType=PID  PIDForm=Parallel  TimeDomain=continuous-time  DiscreteTs=0.1  TuningTs=0.2  UseTuningTs=off  IntegratorFormula=Forward Euler  FilterFormula=Forward Euler  ContinuousTs=0.02  Bandwidth=0.5*2*pi  UseExternalWC=off  TargetPM=60  UseExternalPM=off  UseExternalAchievedPM=off  ExperimentMode=Superposition  PlantType=Integrating  PlantSign=Positive  AmpSine=1  UseExternalAmpSine=off  UseExternalFRD=off  UseExternalU0=off  UseCompanion=off  NotDeployTuningModule=off  UsePLCCoder=off  OutputMode=control action + perturbation  BlockDataType=double  UseConnectedPID=on  blockpath=[]  tunedP=0  tunedI=0  tunedD=0  tunedN=100  tunedPM=0  EstimationWindowSize=3  UseExternalTuningParams=off  SingleMultiRateVariant=SingleSamplingRate  NumEstimationPeriods=4  NumSettlingPeriods=2  NumOfPRBSPeriod=1  PRBSSignalOrder=12  ExperimentModeVariant=VariantSuperimposed  OutputChoice=VariantCandD  ConvergenceCalcVariant=ConvSuperpositionPRBSVariant
      settings: LibrarySourceBlock=slctrlblks/Autotuning/Closed-Loop PID Autotuner
  Constant : Constant  Value=custom_ff
  Constant1 : Constant
  Constant2 : Constant  Value=0
  Demux : Demux  Outputs=3
  Discrete Derivative : simulink/Discrete/Discrete Derivative  gainval=1.0  ICPrevScaledInput=0.0  OutMin=[]  OutMax=[]  OutDataType=fixdt(1, 16)  OutScaling=2^-10  DoSatur=off
  Discrete Derivative1 : simulink/Discrete/Discrete Derivative  gainval=1.0  ICPrevScaledInput=0.0  OutMin=[]  OutMax=[]  OutDataType=fixdt(1, 16)  OutScaling=2^-10  DoSatur=off
  Discrete Derivative2 : simulink/Discrete/Discrete Derivative  gainval=1.0  ICPrevScaledInput=0.0  OutMin=[]  OutMax=[]  OutDataType=fixdt(1, 16)  OutScaling=2^-10  DoSatur=off
  Discrete-Time Integrator1 : DiscreteIntegrator  SampleTime=1/1000  LimitOutput=on  UpperSaturationLimit=MC_RR_INT_LIM  LowerSaturationLimit=-MC_RR_INT_LIM  ICPrevOutput=DiscIntNeverNeededParam  ICPrevScaledInput=DiscIntNeverNeededParam
  Discrete-Time Integrator2 : DiscreteIntegrator  SampleTime=1/1000  LimitOutput=on  UpperSaturationLimit=MC_PR_INT_LIM  LowerSaturationLimit=-MC_PR_INT_LIM  ICPrevOutput=DiscIntNeverNeededParam  ICPrevScaledInput=DiscIntNeverNeededParam
  Discrete-Time Integrator3 : DiscreteIntegrator  SampleTime=1/1000  LimitOutput=on  UpperSaturationLimit=MC_YR_INT_LIM  LowerSaturationLimit=-MC_YR_INT_LIM  ICPrevOutput=DiscIntNeverNeededParam  ICPrevScaledInput=DiscIntNeverNeededParam
  Display : Display
  Display1 : Display
  Gain : Gain  Gain=MC_PITCHRATE_P
  Gain1 : Gain  Gain=MC_PITCHRATE_I
  Gain10 : Gain  Gain=MC_PITCHRATE_K
  Gain11 : Gain  Gain=MC_YAWRATE_K
  Gain12 : Gain  Gain=MC_ROLLRATE_K
  Gain13 : Gain  Gain=MC_YAWRATE_K
  Gain14 : Gain  Gain=MC_PITCHRATE_K
  Gain16 : Gain  Gain=MC_PITCHRATE_FF
  Gain17 : Gain  Gain=tau
  Gain2 : Gain  Gain=MC_PITCHRATE_D
  Gain3 : Gain  Gain=MC_YAWRATE_P
  Gain4 : Gain  Gain=MC_YAWRATE_I
  Gain5 : Gain  Gain=MC_YAWRATE_D
  Gain6 : Gain  Gain=MC_ROLLRATE_P
  Gain7 : Gain  Gain=MC_ROLLRATE_I
  Gain8 : Gain  Gain=MC_ROLLRATE_D
  Gain9 : Gain  Gain=MC_ROLLRATE_K
  LTI System2 : cstblocks/LTI System  sys=c2d(tf(1,[IMU_GYRO_CUTOFF 1]),1/1000)  IC=[]  PadeOrder=0
  LTI System3 : cstblocks/LTI System  sys=c2d(tf(1,[IMU_GYRO_CUTOFF 1]),1/1000)  IC=[]  PadeOrder=0
  LTI System4 : cstblocks/LTI System  sys=c2d(tf(1,[IMU_GYRO_CUTOFF 1]),1/1000)  IC=[]  PadeOrder=0
  LTI System5 : cstblocks/LTI System  sys=c2d(tf(1,[IMU_DGYRO_CUTOFF 1]),1/1000)  IC=[]  PadeOrder=0
  LTI System6 : cstblocks/LTI System  sys=c2d(tf(1,[IMU_DGYRO_CUTOFF 1]),1/1000)  IC=[]  PadeOrder=0
  LTI System7 : cstblocks/LTI System  sys=c2d(tf(1,[IMU_DGYRO_CUTOFF 1]),1/1000)  IC=[]  PadeOrder=0
  Manual Switch : ManualSwitch
  Mux2 : Mux  Inputs=3
  Sum{,1..2,4} (4 alike) : Sum  Inputs=|+-
  Sum3 : Sum  Inputs=|++
  Switch : Switch  Criteria=u2 > Threshold  SaturateOnIntegerOverflow=off  InputSameDT=off
  Delta S.P : Outport
  wires:
  dtheta_sp/1 -> [q_sp]
  LTI System6/1 -> Discrete Derivative1/1
  Sum/1 -> Gain10/1
  Discrete-Time Integrator2/1 -> Gain1/1
  Gain3/1 -> Add1/1
  Gain4/1 -> Add1/2
  Gain5/1 -> Add1/3
  Discrete-Time Integrator3/1 -> Gain4/1
  Sum1/1 -> Gain11/1
  LTI System7/1 -> Discrete Derivative2/1
  [r] -> Gain13/1, Sum1/2  "Feedback"
  [r_sp] -> Sum1/1  "Setpoint"
  Mux2/1 -> Delta S.P/1
  Gain6/1 -> Add2/1
  Gain7/1 -> Add2/2
  Gain8/1 -> Add2/3
  Discrete-Time Integrator1/1 -> Gain7/1
  Sum2/1 -> Gain9/1
  LTI System5/1 -> Discrete Derivative/1
  [p_sp] -> Sum2/1  "Setpoint"
  [q_sp] -> Sum4/1, Switch/3, Sum/1  "Setpoint"
  [p] -> Gain12/1, Sum2/2  "Feedback"
  [q] -> LTI System6/1, Closed-Loop PID Autotuner/2, Sum3/2, Sum/2  "Feedback"
  Add1/1 -> Mux2/3
  Discrete Derivative/1 -> Gain8/1
  Discrete Derivative1/1 -> Gain17/1, Gain14/1
  Discrete Derivative2/1 -> Gain5/1
  Gain9/1 -> Discrete-Time Integrator1/1, Gain6/1
  Gain10/1 -> Discrete-Time Integrator2/1, Gain/1
  Gain11/1 -> Discrete-Time Integrator3/1, Gain3/1
  Gain12/1 -> LTI System5/1
  Gain13/1 -> LTI System7/1
  Gyro/1 -> Demux/1
  dpsi_sp/1 -> [r_sp]
  dphi_sp/1 -> [p_sp]
  Add2/1 -> Mux2/1
  Demux/3 -> [r]
  Demux/2 -> [q]
  Demux/1 -> [p]
  Gain2/1 -> Add/4
  Gain1/1 -> Add/3
  Gain/1 -> Add/2
  Gain16/1 -> Add/1
  Gain17/1 -> Sum3/1
  Switch/1 -> Gain16/1
  Sum4/1 -> Switch/1
  Constant/1 -> Switch/2
  Sum3/1 -> Sum4/2
  Gain14/1 -> Gain2/1
  Add/1 -> Closed-Loop PID Autotuner/1
  Closed-Loop PID Autotuner/1 -> Mux2/2
  Closed-Loop PID Autotuner/2 -> Display/1
  Closed-Loop PID Autotuner/3 -> Display1/1
  Constant2/1 -> Manual Switch/1
  Constant1/1 -> Manual Switch/2
  Manual Switch/1 -> Closed-Loop PID Autotuner/3

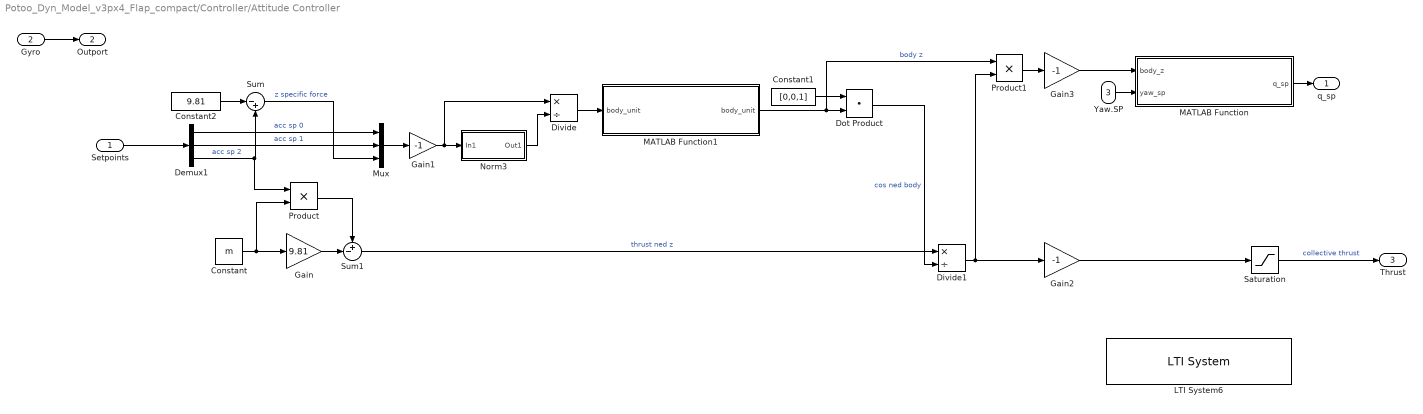
== system Potoo_Dyn_Model_v3px4_Flap_compact/Controller/Attitude Controller ==
  Setpoints : Inport
  Gyro : Inport  Port=2
  Yaw.SP : Inport  Port=3
  Constant : Constant  Value=m
  Constant1 : Constant  Value=[0,0,1]
  Constant2 : Constant  Value=9.81
  Demux1 : Demux  Outputs=3
  Divide : Product  Inputs=*/
  Divide1 : Product  Inputs=*/
  Dot Product : DotProduct  OutDataTypeStr=Inherit: Inherit via internal rule
  Gain : Gain  Gain=9.81
  Gain1 : Gain  Gain=-1
  Gain2 : Gain  Gain=-1
  Gain3 : Gain  Gain=-1
  LTI System6 : cstblocks/LTI System  sys=ss(-10,1,10,0)  IC=m*.981  PadeOrder=0
  MATLAB Function : MATLAB Function  TreatAsAtomicUnit=on
  MATLAB Function1 : MATLAB Function  TreatAsAtomicUnit=on
  Mux : Mux  Inputs=3
  Norm3 : Subsystem
      mask Display: disp('Norm')
  Product : Product
  Product1 : Product
  Saturation : Saturate  UpperLimit=150  LowerLimit=0
  Sum : Sum  Inputs=|-+
  Sum1 : Sum  Inputs=+-|
  q_sp : Outport
  Outport : Outport  Port=2
  Thrust : Outport  Port=3
  wires:
  Setpoints/1 -> Demux1/1
  Gyro/1 -> Outport/1
  Norm3/1(Out1) -> Divide/2
  Constant/1 -> Product/2, Gain/1
  Sum/1 -> Mux/3  "z specific force"
  Divide1/1 -> Product1/2, Gain2/1
  MATLAB Function/1(q_sp) -> q_sp/1
  Yaw.SP/1 -> MATLAB Function/2(yaw_sp)
  Divide/1 -> MATLAB Function1/1("body_unit ")
  Dot Product/1 -> Divide1/2  "cos ned body"
  Demux1/1 -> Mux/1  "acc sp 0"
  Demux1/2 -> Mux/2  "acc sp 1"
  Mux/1 -> Gain1/1
  Constant2/1 -> Sum/1
  Gain1/1 -> Divide/1, Norm3/1(In1)
  Demux1/3 -> Product/1, Sum/2  "acc sp 2"
  Gain/1 -> Sum1/2
  Product/1 -> Sum1/1
  Sum1/1 -> Divide1/1  "thrust ned z"
  Constant1/1 -> Dot Product/1
  Product1/1 -> Gain3/1
  MATLAB Function1/1(body_unit) -> Product1/1, Dot Product/2  "body z"
  Saturation/1 -> Thrust/1  "collective thrust"
  Gain2/1 -> Saturation/1
  Gain3/1 -> MATLAB Function/1(body_z)

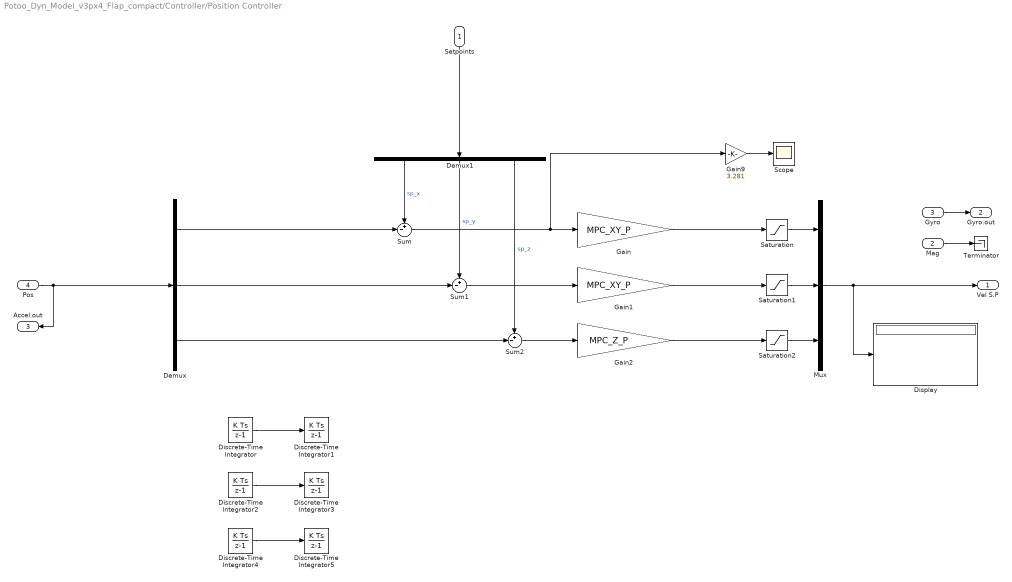
== system Potoo_Dyn_Model_v3px4_Flap_compact/Controller/Position Controller ==
  Setpoints : Inport
  Mag : Inport  Port=2
  Gyro : Inport  Port=3
  Pos : Inport  Port=4
  Demux : Demux  Outputs=3
  Demux1 : Demux  Outputs=3
  Discrete-Time Integrator : DiscreteIntegrator  SampleTime=Tmech  ICPrevOutput=DiscIntNeverNeededParam  ICPrevScaledInput=DiscIntNeverNeededParam
  Discrete-Time Integrator1 : DiscreteIntegrator  SampleTime=-1  ICPrevOutput=DiscIntNeverNeededParam  ICPrevScaledInput=DiscIntNeverNeededParam
  Discrete-Time Integrator2 : DiscreteIntegrator  SampleTime=Tmech  ICPrevOutput=DiscIntNeverNeededParam  ICPrevScaledInput=DiscIntNeverNeededParam
  Discrete-Time Integrator3 : DiscreteIntegrator  SampleTime=-1  ICPrevOutput=DiscIntNeverNeededParam  ICPrevScaledInput=DiscIntNeverNeededParam
  Discrete-Time Integrator4 : DiscreteIntegrator  SampleTime=Tmech  LimitOutput=on  UpperSaturationLimit=1  ICPrevOutput=DiscIntNeverNeededParam  ICPrevScaledInput=DiscIntNeverNeededParam
  Discrete-Time Integrator5 : DiscreteIntegrator  InitialCondition=-5*.3048  SampleTime=-1  LimitOutput=on  UpperSaturationLimit=0  ICPrevOutput=DiscIntNeverNeededParam  ICPrevScaledInput=DiscIntNeverNeededParam
  Display : Display
  Gain : Gain  Gain=MPC_XY_P
  Gain1 : Gain  Gain=MPC_XY_P
  Gain2 : Gain  Gain=MPC_Z_P
  Gain9 : Gain  Gain=3.281
  Mux : Mux  Inputs=3
  Saturation : Saturate  UpperLimit=MPC_XY_VEL_MAX  LowerLimit=-MPC_XY_VEL_MAX
  Saturation1 : Saturate  UpperLimit=MPC_XY_VEL_MAX  LowerLimit=-MPC_XY_VEL_MAX
  Saturation2 : Saturate  UpperLimit=MPC_Z_VEL_MAX_DOWN  LowerLimit=-MPC_Z_VEL_MAX_UP
  Scope : Scope
  Sum : Sum  Inputs=+-|
  Sum1 : Sum  Inputs=+-|
  Sum2 : Sum  Inputs=+-|
  Terminator : Terminator
  Vel S.P : Outport
  Gyro.out : Outport  Port=2
  Accel.out : Outport  Port=3
  wires:
  Mag/1 -> Terminator/1
  Gyro/1 -> Gyro.out/1
  Discrete-Time Integrator/1 -> Discrete-Time Integrator1/1
  Demux1/1 -> Sum/1  "sp_x"
  Demux1/2 -> Sum1/1  "sp_y"
  Demux1/3 -> Sum2/1  "sp_z"
  Sum1/1 -> Gain1/1
  Sum2/1 -> Gain2/1
  Gain/1 -> Saturation/1
  Gain1/1 -> Saturation1/1
  Gain2/1 -> Saturation2/1
  Saturation2/1 -> Mux/3
  Saturation1/1 -> Mux/2
  Saturation/1 -> Mux/1
  Mux/1 -> Display/1, Vel S.P/1
  Pos/1 -> Demux/1, Accel.out/1
  Discrete-Time Integrator2/1 -> Discrete-Time Integrator3/1
  Discrete-Time Integrator4/1 -> Discrete-Time Integrator5/1
  Setpoints/1 -> Demux1/1
  Demux/1 -> Sum/2
  Demux/2 -> Sum1/2
  Demux/3 -> Sum2/2
  Sum/1 -> Gain9/1, Gain/1
  Gain9/1 -> Scope/1

== system Potoo_Dyn_Model_v3px4_Flap_compact/Controller/Subsystem ==
  acc : Inport
  rate : Inport  Port=2
  AHRS : mspfiltlib/AHRS  DispRefFrame=NED  DecimationFactor=1  InitialProcessNoise=ahrsfilter.defaultProcessNoise  OrientationFormat=quaternion  SimulateUsing=Code generation  AccelerometerNoise=0.0001924722  GyroscopeNoise=9.1385e-5  MagnetometerNoise=0.1  GyroscopeDriftNoise=3.0462e-13  LinearAccelerationNoise=0.0096236100000000012  MagneticDisturbanceNoise=0.5  LinearAccelerationDecayFactor=0.5  MagneticDisturbanceDecayFactor=0.5  ExpectedMagneticFieldStrength=50
  Add : Sum  Inputs=+-
  IMU1 : mspsensorlib/IMU  DispRefFrame=NED  TemperaturePort=off  Temperature=25  MagneticFieldPort=off  MagneticFieldNED=[ 27.5550, -2.4169, -16.0849 ]  MagneticFieldENU=[ -2.4169, 27.5550, 16.0849 ]  SeedDouble=50  SimulateUsing=Code generation  AccelParamsMeasurementRange=4*9.81  AccelParamsResolution=1/(8192*9.81)  AccelParamsConstantBias=[0 0 0]  AccelParamsAxesMisalignment=[0 0 0]  AccelParamsNoiseDensity=1377e-6*[0 0 0]  AccelParamsBiasInstability=[0 0 0]  AccelParamsBiasInstabilityNumerator=fractalcoef().Numerator  AccelParamsBiasInstabilityDenominator=fractalcoef().Denominator  AccelParamsRandomWalk=[0 0 0]  AccelParamsNoiseType=double-sided  AccelParamsTemperatureBias=[0 0 0]  AccelParamsTemperatureScaleFactor=[0 0 0]  GyroParamsMeasurementRange=17.4532  GyroParamsResolution=1/3752  GyroParamsConstantBias=[0 0 0]  GyroParamsAxesMisalignment=0  GyroParamsAccelerationBias=[0 0 0]  GyroParamsNoiseDensity=[0 0 0].*0.000  GyroParamsBiasInstability=[0 0 0]  GyroParamsBiasInstabilityNumerator=fractalcoef().Numerator  GyroParamsBiasInstabilityDenominator=fractalcoef().Denominator  GyroParamsRandomWalk=[0 0 0]  GyroParamsNoiseType=double-sided  GyroParamsTemperatureBias=[0 0 0]  GyroParamsTemperatureScaleFactor=[0 0 0]  MagParamsMeasurementRange=1600  MagParamsResolution=0.3  MagParamsConstantBias=0  MagParamsAxesMisalignment=[0 0 0]  MagParamsNoiseDensity=[0 0 0]  MagParamsBiasInstability=[0 0 0]  MagParamsBiasInstabilityNumerator=fractalcoef().Numerator  MagParamsBiasInstabilityDenominator=fractalcoef().Denominator  MagParamsRandomWalk=[0 0 0]  MagParamsNoiseType=double-sided  MagParamsTemperatureBias=[0 0 0]  MagParamsTemperatureScaleFactor=[0 0 0]
  Integrate Angular Velocity : MATLAB Function  TreatAsAtomicUnit=on  mask{rate=1/1000}
      mask prompts: rate "Sample Rate"
  Manual Switch : ManualSwitch
  Terminator2 : Terminator
  Terminator3 : Terminator
  Transpose3 : Math  Operator=transpose
  Transpose4 : Math  Operator=transpose
  Transpose5 : Math  Operator=transpose
  Zero-Order Hold : ZeroOrderHold  SampleTime=-1
  Zero-Order Hold1 : ZeroOrderHold  SampleTime=-1
  accel : Outport
  gyro : Outport  Port=2
  wires:
  acc/1 -> Zero-Order Hold/1
  AHRS/1 -> Terminator2/1
  Add/1 -> Terminator3/1  "error"
  Transpose4/1 -> IMU1/1
  AHRS/2 -> Transpose5/1
  rate/1 -> Zero-Order Hold1/1  "angular rate"
  Integrate Angular Velocity/1(q) -> IMU1/3
  IMU1/3 -> AHRS/3
  Transpose5/1 -> Manual Switch/1, Add/1  "gyro"
  IMU1/1 -> accel/1, AHRS/1
  Transpose3/1 -> Integrate Angular Velocity/1(av), IMU1/2
  IMU1/2 -> AHRS/2
  Manual Switch/1 -> gyro/1
  Zero-Order Hold/1 -> Transpose4/1
  Zero-Order Hold1/1 -> Manual Switch/2, Add/2, Transpose3/1

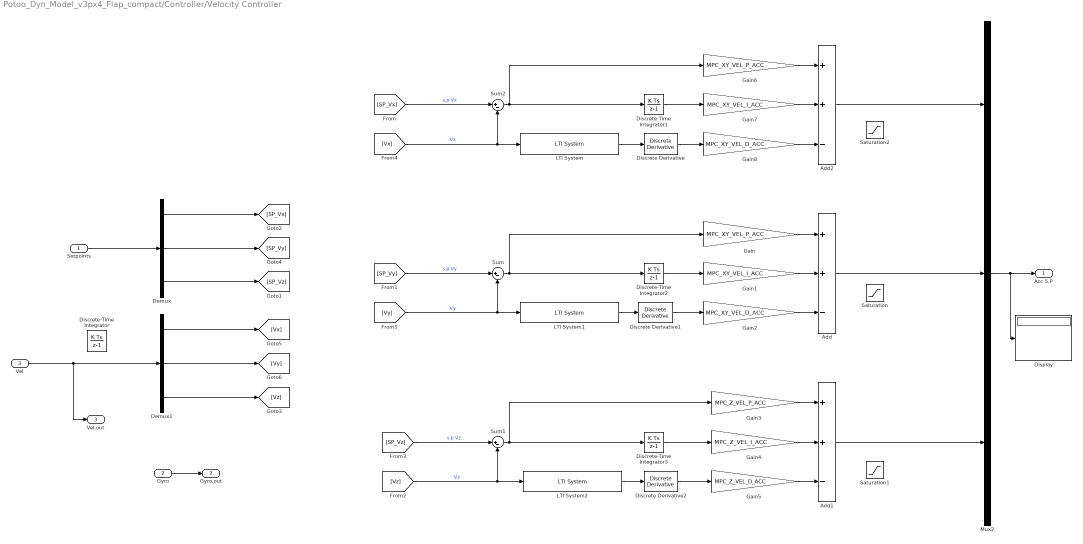
== system Potoo_Dyn_Model_v3px4_Flap_compact/Controller/Velocity Controller ==
  Setpoints : Inport
  Gyro : Inport  Port=2
  Vel : Inport  Port=3
  Add : Sum  Inputs=++-
  Add1 : Sum  Inputs=++-
  Add2 : Sum  Inputs=++-
  Demux : Demux  Outputs=3
  Demux1 : Demux  Outputs=3
  Discrete Derivative : simulink/Discrete/Discrete Derivative  gainval=1.0  ICPrevScaledInput=0.0  OutMin=[]  OutMax=[]  OutDataType=fixdt(1, 16)  OutScaling=2^-10  DoSatur=off
  Discrete Derivative1 : simulink/Discrete/Discrete Derivative  gainval=1.0  ICPrevScaledInput=0.0  OutMin=[]  OutMax=[]  OutDataType=fixdt(1, 16)  OutScaling=2^-10  DoSatur=off
  Discrete Derivative2 : simulink/Discrete/Discrete Derivative  gainval=1.0  ICPrevScaledInput=0.0  OutMin=[]  OutMax=[]  OutDataType=fixdt(1, 16)  OutScaling=2^-10  DoSatur=off
  Discrete-Time Integrator{,1..3} (4 alike) : DiscreteIntegrator  SampleTime=Tmech  ICPrevOutput=DiscIntNeverNeededParam  ICPrevScaledInput=DiscIntNeverNeededParam
  Display : Display
  Gain : Gain  Gain=MPC_XY_VEL_P_ACC
  Gain1 : Gain  Gain=MPC_XY_VEL_I_ACC
  Gain2 : Gain  Gain=MPC_XY_VEL_D_ACC
  Gain3 : Gain  Gain=MPC_Z_VEL_P_ACC
  Gain4 : Gain  Gain=MPC_Z_VEL_I_ACC
  Gain5 : Gain  Gain=MPC_Z_VEL_D_ACC
  Gain6 : Gain  Gain=MPC_XY_VEL_P_ACC
  Gain7 : Gain  Gain=MPC_XY_VEL_I_ACC
  Gain8 : Gain  Gain=MPC_XY_VEL_D_ACC
  LTI System : cstblocks/LTI System  sys=c2d(tf(1,[MPC_VELD_LP 1]),Tmech)  IC=[]  PadeOrder=0
  LTI System1 : cstblocks/LTI System  sys=c2d(tf(1,[MPC_VELD_LP 1]),Tmech)  IC=[]  PadeOrder=0
  LTI System2 : cstblocks/LTI System  sys=c2d(tf(1,[MPC_VELD_LP 1]),Tmech)  IC=[]  PadeOrder=0
  Mux2 : Mux  Inputs=3
  Saturation : Saturate  UpperLimit=MPC_TILTMAX_AIR  LowerLimit=-MPC_TILTMAX_AIR
  Saturation1 : Saturate  UpperLimit=MPC_THR_MAX  LowerLimit=0
  Saturation2 : Saturate  UpperLimit=MPC_TILTMAX_AIR  LowerLimit=-MPC_TILTMAX_AIR
  Sum : Sum  Inputs=|+-
  Sum1 : Sum  Inputs=|+-
  Sum2 : Sum  Inputs=|+-
  Acc S.P : Outport
  Gyro.out : Outport  Port=2
  Vel.out : Outport  Port=3
  wires:
  Setpoints/1 -> Demux/1
  Demux/3 -> [SP_Vz]
  Gyro/1 -> Gyro.out/1
  LTI System1/1 -> Discrete Derivative1/1
  Sum/1 -> Discrete-Time Integrator2/1, Gain/1
  Discrete-Time Integrator2/1 -> Gain1/1
  Gain2/1 -> Add/3
  Gain1/1 -> Add/2
  Gain/1 -> Add/1
  Gain3/1 -> Add1/1
  Discrete-Time Integrator3/1 -> Gain4/1
  Sum1/1 -> Discrete-Time Integrator3/1, Gain3/1
  LTI System2/1 -> Discrete Derivative2/1
  [Vz] -> LTI System2/1, Sum1/2  "Vz"
  [SP_Vz] -> Sum1/1  "s.p Vz"
  Mux2/1 -> Display/1, Acc S.P/1
  Gain6/1 -> Add2/1
  Gain7/1 -> Add2/2
  Gain8/1 -> Add2/3
  Discrete-Time Integrator1/1 -> Gain7/1
  Sum2/1 -> Discrete-Time Integrator1/1, Gain6/1
  LTI System/1 -> Discrete Derivative/1
  Demux/1 -> [SP_Vx]
  Demux/2 -> [SP_Vy]
  [SP_Vx] -> Sum2/1  "s.p Vx"
  [SP_Vy] -> Sum/1  "s.p Vy"
  Demux1/1 -> [Vx]
  [Vx] -> LTI System/1, Sum2/2  "Vx"
  Demux1/2 -> [Vy]
  [Vy] -> LTI System1/1, Sum/2  "Vy"
  Discrete Derivative/1 -> Gain8/1
  Discrete Derivative1/1 -> Gain2/1
  Discrete Derivative2/1 -> Gain5/1
  Vel/1 -> Demux1/1, Vel.out/1
  Demux1/3 -> [Vz]
  Add2/1 -> Mux2/1
  Add/1 -> Mux2/2
  Add1/1 -> Mux2/3
  Gain4/1 -> Add1/2
  Gain5/1 -> Add1/3
